simulink model "Tandem4Servers10000"  (R2023a)
settings: Solver=VariableStepAuto  StartTime=0.0  StopTime=100  RelTol=1e-3
undefined symbols (not defined in the file or in its folder): m, n
libraries: simulink x2
settings Model: PauseTimes=53  Creator=pratyaksh  LastModifiedBy=pratyaksh

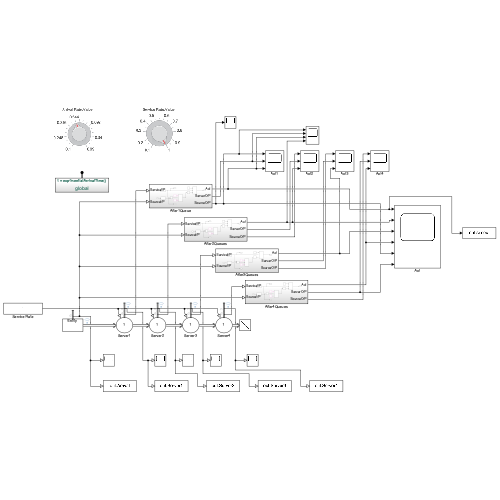
[thumbnail: Simulink's stored preview of the top-level diagram]
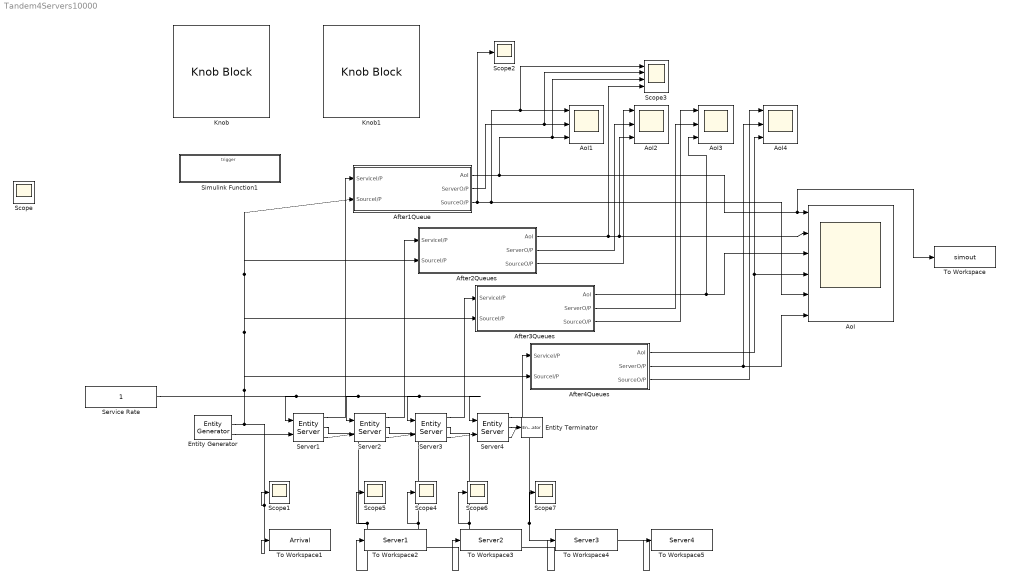
== system Tandem4Servers10000 ==
  After1Queue : Subsystem
  After2Queues : Subsystem
  After3Queues : Subsystem
  After4Queues : Subsystem
  AoI : Scope  NumInputPorts=6
  AoI{1..4} (4 alike) : Scope  NumInputPorts=3
  Entity Generator : EntityGenerator  OutputPortMessageModes=n,m  TimeSource=MATLAB action  Period=7  IntergenerationTimeAction=|  GenerateEntityAtSimulationStart=off  AttributeInitialValue=0  NumberEntitiesDeparted=on  EntityType=Structured  EntityTypeName=Entity
      | T = exponentialArrivalTime;   % fixed intergeneration time
      | N = 10000;   % number of entities generated
      | persistent nr;
      | if isempty(nr)
      |   nr = 1;
      | end
      | 
      | if nr <= N
      |   dt = T;
      | else
      |   dt = inf;
      | end
      | nr = nr + 1;
      settings: OutputPortMap=o0,o3
  Entity Terminator : EntityTerminator  InputPortMessageModes=m
  Knob : KnobBlock  ScaleMin=0.10000000000000001  ScaleMax=0.99
  Knob1 : KnobBlock  ScaleMin=0.10000000000000001  ScaleMax=1
  Scope{,1..2,4..7} (7 alike) : Scope
  Scope3 : Scope  NumInputPorts=4
  Server1 : EntityServer  InputPortMessageModes=n,m  OutputPortMessageModes=n,n,m  Capacity=1  ServiceTimeSource=Signal port  ServiceTimeAction=|  NumberEntitiesDeparted=on  NumberEntitiesInBlock=on
      | persistent rngInit;
      | if isempty(rngInit)
      |     seed = 12345;
      |     rng(seed);
      |     rngInit = true;
      | end
      | 
      | % Pattern: Exponential distribution
      | mu = 1;
      | dt = -mu * log(1 - rand());
      settings: InputPortMap=u0,u2  OutputPortMap=o0,o1,o9
  Server2 : EntityServer  InputPortMessageModes=n,m  OutputPortMessageModes=n,n,m  Capacity=1  ServiceTimeSource=Signal port  ServiceTimeAction=|  NumberEntitiesDeparted=on  NumberEntitiesInBlock=on
      | persistent rngInit;
      | if isempty(rngInit)
      |     seed = 12345;
      |     rng(seed);
      |     rngInit = true;
      | end
      | 
      | % Pattern: Exponential distribution
      | mu = 1;
      | dt = -mu * log(1 - rand());
      settings: InputPortMap=u0,u2  OutputPortMap=o0,o1,o9
  Server3 : EntityServer  InputPortMessageModes=n,m  OutputPortMessageModes=n,n,m  Capacity=1  ServiceTimeSource=Signal port  ServiceTimeAction=|  NumberEntitiesDeparted=on  NumberEntitiesInBlock=on
      | persistent rngInit;
      | if isempty(rngInit)
      |     seed = 12345;
      |     rng(seed);
      |     rngInit = true;
      | end
      | 
      | % Pattern: Exponential distribution
      | mu = 1;
      | dt = -mu * log(1 - rand());
      settings: InputPortMap=u0,u2  OutputPortMap=o0,o1,o9
  Server4 : EntityServer  InputPortMessageModes=n,m  OutputPortMessageModes=n,n,m  Capacity=1  ServiceTimeSource=Signal port  ServiceTimeAction=|  NumberEntitiesDeparted=on  NumberEntitiesInBlock=on
      | persistent rngInit;
      | if isempty(rngInit)
      |     seed = 12345;
      |     rng(seed);
      |     rngInit = true;
      | end
      | 
      | % Pattern: Exponential distribution
      | mu = 1;
      | dt = -mu * log(1 - rand());
      settings: InputPortMap=u0,u2  OutputPortMap=o0,o1,o9
  Service Rate : Constant  SampleTime=-1
  Simulink Function1 : Subsystem  TreatAsAtomicUnit=on
  To Workspace : ToWorkspace  VariableName=simout  SampleTime=-1
      settings: MaxDataPoints=2  Save2DSignal=2-D array (concatenate along first dimension)
  To Workspace1 : ToWorkspace  VariableName=Arrival  SaveFormat=Timeseries  SampleTime=-1
  To Workspace2 : ToWorkspace  VariableName=Server1  SaveFormat=Timeseries  SampleTime=-1
      settings: Save2DSignal=2-D array (concatenate along first dimension)
  To Workspace3 : ToWorkspace  VariableName=Server2  SaveFormat=Timeseries  SampleTime=-1
      settings: Save2DSignal=2-D array (concatenate along first dimension)
  To Workspace4 : ToWorkspace  VariableName=Server3  SaveFormat=Timeseries  SampleTime=-1
      settings: Save2DSignal=2-D array (concatenate along first dimension)
  To Workspace5 : ToWorkspace  VariableName=Server4  SaveFormat=Timeseries  SampleTime=-1
      settings: Save2DSignal=2-D array (concatenate along first dimension)
  wires:
  Service Rate/1 -> Server1/1, Server2/1, Server3/1, Server4/1
  Entity Generator/2 -> Server1/2
  Server3/3 -> Server4/2
  Server4/3 -> Entity Terminator/1
  Server1/3 -> Server2/2
  Server2/3 -> Server3/2
  Entity Generator/1 -> After4Queues/2(SourceI/P), After2Queues/2(SourceI/P), After1Queue/2(SourceI/P), After3Queues/2(SourceI/P), To Workspace1/1, Scope1/1
  Server4/1 -> After4Queues/1(ServiceI/P)
  Server3/1 -> After3Queues/1(ServiceI/P)
  Server2/1 -> After2Queues/1(ServiceI/P)
  Server1/1 -> After1Queue/1(ServiceI/P)
  After2Queues/1(AoI) -> Scope3/4, AoI/2, AoI2/3
  After3Queues/1(AoI) -> AoI/3, AoI3/3
  After4Queues/1(AoI) -> AoI4/3, AoI/4
  After1Queue/3(SourceO/P) -> Scope2/1, Scope3/1, AoI1/1, AoI/5
  After4Queues/2(ServerO/P) -> AoI/6, AoI4/2
  After1Queue/2(ServerO/P) -> Scope3/2, AoI1/2
  After2Queues/3(SourceO/P) -> AoI2/1
  After2Queues/2(ServerO/P) -> AoI2/2
  After3Queues/3(SourceO/P) -> AoI3/1
  After3Queues/2(ServerO/P) -> AoI3/2
  After4Queues/3(SourceO/P) -> AoI4/1
  After1Queue/1(AoI) -> Scope3/3, AoI1/3, To Workspace/1, AoI/1
  Server2/2 -> To Workspace3/1, Scope4/1
  Server3/2 -> To Workspace4/1, Scope6/1
  Server4/2 -> To Workspace5/1, Scope7/1
  Server1/2 -> To Workspace2/1, Scope5/1

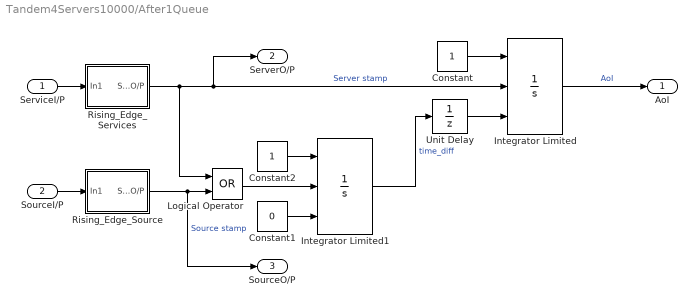
== system Tandem4Servers10000/After1Queue ==
  ServiceI/P : Inport
  SourceI/P : Inport  Port=2
  Constant : Constant
  Constant1 : Constant  Value=0
  Constant2 : Constant
  Integrator Limited : Integrator  ExternalReset=rising  InitialConditionSource=external  LimitOutput=on  UpperSaturationLimit=1000  LowerSaturationLimit=0
  Integrator Limited1 : Integrator  ExternalReset=rising  InitialConditionSource=external  LimitOutput=on  UpperSaturationLimit=1000  LowerSaturationLimit=0
  Logical Operator : Logic  Operator=OR  AllPortsSameDT=off  OutDataTypeStr=boolean
  Rising_Edge_Services : Subsystem
  Rising_Edge_Source : Subsystem
  Unit Delay : UnitDelay  SampleTime=-1  HasFrameUpgradeWarning=on
  AoI : Outport
  ServerO/P : Outport  Port=2
  SourceO/P : Outport  Port=3
  wires:
  Unit Delay/1 -> Integrator Limited/3
  Logical Operator/1 -> Integrator Limited1/2
  Rising_Edge_Source/1(SourceO/P) -> SourceO/P/1, Logical Operator/2  "Source stamp"
  Integrator Limited1/1 -> Unit Delay/1  "time_diff"
  Constant1/1 -> Integrator Limited1/3
  Rising_Edge_Services/1(ServerO/P) -> ServerO/P/1, Integrator Limited/2, Logical Operator/1  "Server stamp"
  Constant2/1 -> Integrator Limited1/1
  SourceI/P/1 -> Rising_Edge_Source/1(In1)
  ServiceI/P/1 -> Rising_Edge_Services/1(In1)
  Constant/1 -> Integrator Limited/1
  Integrator Limited/1 -> AoI/1  "AoI"

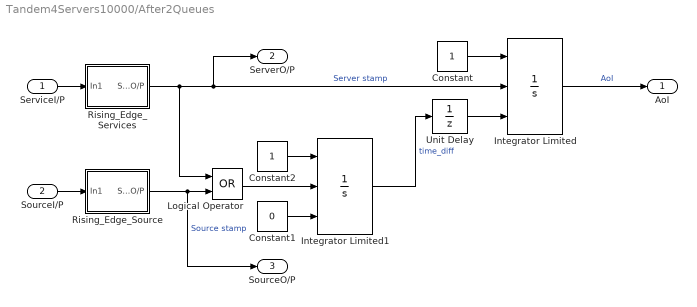
== system Tandem4Servers10000/After2Queues ==
  ServiceI/P : Inport
  SourceI/P : Inport  Port=2
  Constant : Constant
  Constant1 : Constant  Value=0
  Constant2 : Constant
  Integrator Limited : Integrator  ExternalReset=rising  InitialConditionSource=external  LimitOutput=on  UpperSaturationLimit=1000  LowerSaturationLimit=0
  Integrator Limited1 : Integrator  ExternalReset=rising  InitialConditionSource=external  LimitOutput=on  UpperSaturationLimit=1000  LowerSaturationLimit=0
  Logical Operator : Logic  Operator=OR  AllPortsSameDT=off  OutDataTypeStr=boolean
  Rising_Edge_Services : Subsystem
  Rising_Edge_Source : Subsystem
  Unit Delay : UnitDelay  SampleTime=-1  HasFrameUpgradeWarning=on
  AoI : Outport
  ServerO/P : Outport  Port=2
  SourceO/P : Outport  Port=3
  wires:
  Unit Delay/1 -> Integrator Limited/3
  Logical Operator/1 -> Integrator Limited1/2
  Rising_Edge_Source/1(SourceO/P) -> SourceO/P/1, Logical Operator/2  "Source stamp"
  Integrator Limited1/1 -> Unit Delay/1  "time_diff"
  Constant1/1 -> Integrator Limited1/3
  Rising_Edge_Services/1(ServerO/P) -> ServerO/P/1, Integrator Limited/2, Logical Operator/1  "Server stamp"
  Constant2/1 -> Integrator Limited1/1
  SourceI/P/1 -> Rising_Edge_Source/1(In1)
  ServiceI/P/1 -> Rising_Edge_Services/1(In1)
  Constant/1 -> Integrator Limited/1
  Integrator Limited/1 -> AoI/1  "AoI"

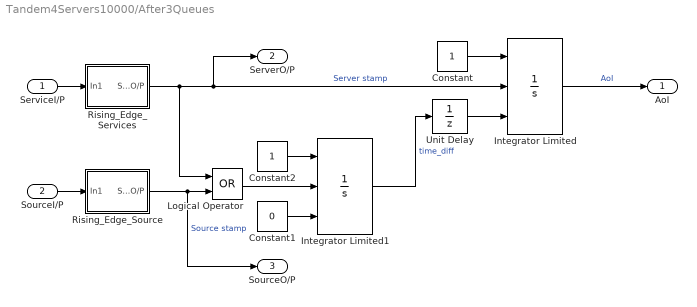
== system Tandem4Servers10000/After3Queues ==
  ServiceI/P : Inport
  SourceI/P : Inport  Port=2
  Constant : Constant
  Constant1 : Constant  Value=0
  Constant2 : Constant
  Integrator Limited : Integrator  ExternalReset=rising  InitialConditionSource=external  LimitOutput=on  UpperSaturationLimit=1000  LowerSaturationLimit=0
  Integrator Limited1 : Integrator  ExternalReset=rising  InitialConditionSource=external  LimitOutput=on  UpperSaturationLimit=1000  LowerSaturationLimit=0
  Logical Operator : Logic  Operator=OR  AllPortsSameDT=off  OutDataTypeStr=boolean
  Rising_Edge_Services : Subsystem
  Rising_Edge_Source : Subsystem
  Unit Delay : UnitDelay  SampleTime=-1  HasFrameUpgradeWarning=on
  AoI : Outport
  ServerO/P : Outport  Port=2
  SourceO/P : Outport  Port=3
  wires:
  Unit Delay/1 -> Integrator Limited/3
  Logical Operator/1 -> Integrator Limited1/2
  Rising_Edge_Source/1(SourceO/P) -> SourceO/P/1, Logical Operator/2  "Source stamp"
  Integrator Limited1/1 -> Unit Delay/1  "time_diff"
  Constant1/1 -> Integrator Limited1/3
  Rising_Edge_Services/1(ServerO/P) -> ServerO/P/1, Integrator Limited/2, Logical Operator/1  "Server stamp"
  Constant2/1 -> Integrator Limited1/1
  SourceI/P/1 -> Rising_Edge_Source/1(In1)
  ServiceI/P/1 -> Rising_Edge_Services/1(In1)
  Constant/1 -> Integrator Limited/1
  Integrator Limited/1 -> AoI/1  "AoI"

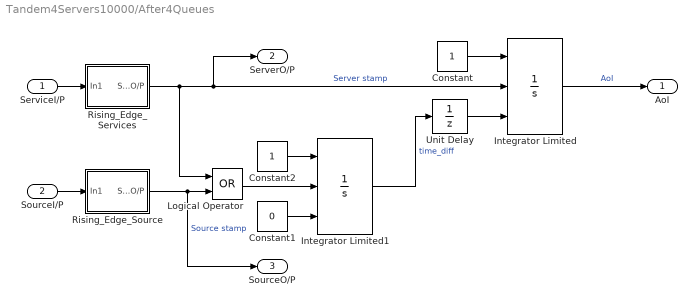
== system Tandem4Servers10000/After4Queues ==
  ServiceI/P : Inport
  SourceI/P : Inport  Port=2
  Constant : Constant
  Constant1 : Constant  Value=0
  Constant2 : Constant
  Integrator Limited : Integrator  ExternalReset=rising  InitialConditionSource=external  LimitOutput=on  UpperSaturationLimit=1000  LowerSaturationLimit=0
  Integrator Limited1 : Integrator  ExternalReset=rising  InitialConditionSource=external  LimitOutput=on  UpperSaturationLimit=1000  LowerSaturationLimit=0
  Logical Operator : Logic  Operator=OR  AllPortsSameDT=off  OutDataTypeStr=boolean
  Rising_Edge_Services : Subsystem
  Rising_Edge_Source : Subsystem
  Unit Delay : UnitDelay  SampleTime=-1  HasFrameUpgradeWarning=on
  AoI : Outport
  ServerO/P : Outport  Port=2
  SourceO/P : Outport  Port=3
  wires:
  Unit Delay/1 -> Integrator Limited/3
  Logical Operator/1 -> Integrator Limited1/2
  Rising_Edge_Source/1(SourceO/P) -> SourceO/P/1, Logical Operator/2  "Source stamp"
  Integrator Limited1/1 -> Unit Delay/1  "time_diff"
  Constant1/1 -> Integrator Limited1/3
  Rising_Edge_Services/1(ServerO/P) -> ServerO/P/1, Integrator Limited/2, Logical Operator/1  "Server stamp"
  Constant2/1 -> Integrator Limited1/1
  SourceI/P/1 -> Rising_Edge_Source/1(In1)
  ServiceI/P/1 -> Rising_Edge_Services/1(In1)
  Constant/1 -> Integrator Limited/1
  Integrator Limited/1 -> AoI/1  "AoI"

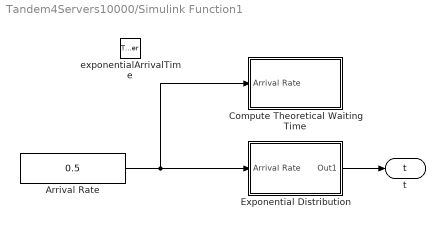
== system Tandem4Servers10000/Simulink Function1 ==
  exponentialArrivalTime : TriggerPort  TriggerType=function-call  IsSimulinkFunction=on  FunctionName=exponentialArrivalTime  VariantControl=Variant
  Arrival Rate : Constant  Value=0.5  SampleTime=-1
  Compute Theoretical Waiting Time : Subsystem
  Exponential Distribution : Subsystem
  t : ArgOut  DisableCoverage=on  ArgumentName=t
  wires:
  Exponential Distribution/1(Out1) -> t/1
  Arrival Rate/1 -> Exponential Distribution/1(Arrival Rate), Compute Theoretical Waiting Time/1(Arrival Rate)

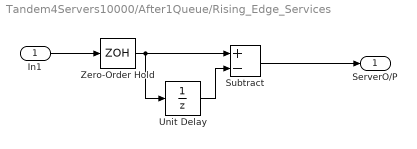
== system Tandem4Servers10000/After1Queue/Rising_Edge_Services ==
  In1 : Inport
  Subtract : Sum  Inputs=+-
  Unit Delay : UnitDelay  SampleTime=-1  HasFrameUpgradeWarning=on
  Zero-Order Hold : ZeroOrderHold  SampleTime=0.005
  ServerO/P : Outport  VectorParamsAs1DForOutWhenUnconnected=off
  wires:
  Zero-Order Hold/1 -> Unit Delay/1, Subtract/1
  Unit Delay/1 -> Subtract/2
  In1/1 -> Zero-Order Hold/1
  Subtract/1 -> ServerO/P/1

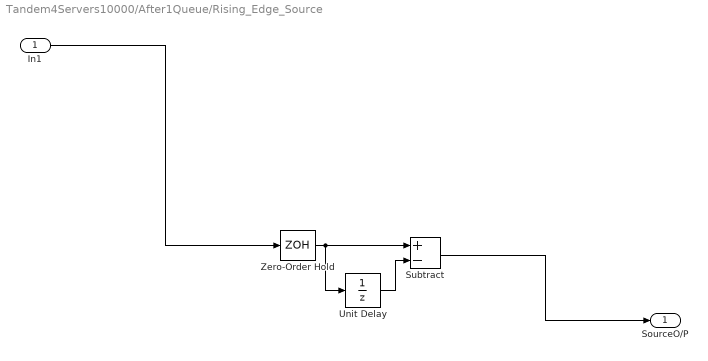
== system Tandem4Servers10000/After1Queue/Rising_Edge_Source ==
  In1 : Inport
  Subtract : Sum  Inputs=+-
  Unit Delay : UnitDelay  SampleTime=-1  HasFrameUpgradeWarning=on
  Zero-Order Hold : ZeroOrderHold  SampleTime=0.005
  SourceO/P : Outport  VectorParamsAs1DForOutWhenUnconnected=off
  wires:
  Zero-Order Hold/1 -> Unit Delay/1, Subtract/1
  Unit Delay/1 -> Subtract/2
  In1/1 -> Zero-Order Hold/1
  Subtract/1 -> SourceO/P/1

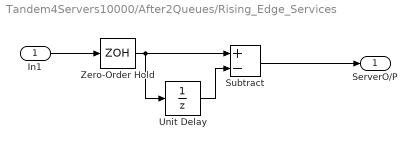
== system Tandem4Servers10000/After2Queues/Rising_Edge_Services ==
  In1 : Inport
  Subtract : Sum  Inputs=+-
  Unit Delay : UnitDelay  SampleTime=-1  HasFrameUpgradeWarning=on
  Zero-Order Hold : ZeroOrderHold  SampleTime=0.005
  ServerO/P : Outport  VectorParamsAs1DForOutWhenUnconnected=off
  wires:
  Zero-Order Hold/1 -> Unit Delay/1, Subtract/1
  Unit Delay/1 -> Subtract/2
  In1/1 -> Zero-Order Hold/1
  Subtract/1 -> ServerO/P/1

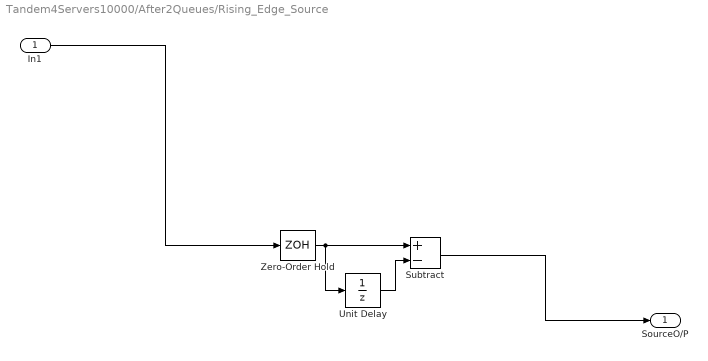
== system Tandem4Servers10000/After2Queues/Rising_Edge_Source ==
  In1 : Inport
  Subtract : Sum  Inputs=+-
  Unit Delay : UnitDelay  SampleTime=-1  HasFrameUpgradeWarning=on
  Zero-Order Hold : ZeroOrderHold  SampleTime=0.005
  SourceO/P : Outport  VectorParamsAs1DForOutWhenUnconnected=off
  wires:
  Zero-Order Hold/1 -> Unit Delay/1, Subtract/1
  Unit Delay/1 -> Subtract/2
  In1/1 -> Zero-Order Hold/1
  Subtract/1 -> SourceO/P/1

== system Tandem4Servers10000/After3Queues/Rising_Edge_Services ==
  In1 : Inport
  Subtract : Sum  Inputs=+-
  Unit Delay : UnitDelay  SampleTime=-1  HasFrameUpgradeWarning=on
  Zero-Order Hold : ZeroOrderHold  SampleTime=0.005
  ServerO/P : Outport  VectorParamsAs1DForOutWhenUnconnected=off
  wires:
  Zero-Order Hold/1 -> Unit Delay/1, Subtract/1
  Unit Delay/1 -> Subtract/2
  In1/1 -> Zero-Order Hold/1
  Subtract/1 -> ServerO/P/1

== system Tandem4Servers10000/After3Queues/Rising_Edge_Source ==
  In1 : Inport
  Subtract : Sum  Inputs=+-
  Unit Delay : UnitDelay  SampleTime=-1  HasFrameUpgradeWarning=on
  Zero-Order Hold : ZeroOrderHold  SampleTime=0.005
  SourceO/P : Outport  VectorParamsAs1DForOutWhenUnconnected=off
  wires:
  Zero-Order Hold/1 -> Unit Delay/1, Subtract/1
  Unit Delay/1 -> Subtract/2
  In1/1 -> Zero-Order Hold/1
  Subtract/1 -> SourceO/P/1

== system Tandem4Servers10000/After4Queues/Rising_Edge_Services ==
  In1 : Inport
  Subtract : Sum  Inputs=+-
  Unit Delay : UnitDelay  SampleTime=-1  HasFrameUpgradeWarning=on
  Zero-Order Hold : ZeroOrderHold  SampleTime=0.005
  ServerO/P : Outport  VectorParamsAs1DForOutWhenUnconnected=off
  wires:
  Zero-Order Hold/1 -> Unit Delay/1, Subtract/1
  Unit Delay/1 -> Subtract/2
  In1/1 -> Zero-Order Hold/1
  Subtract/1 -> ServerO/P/1

== system Tandem4Servers10000/After4Queues/Rising_Edge_Source ==
  In1 : Inport
  Subtract : Sum  Inputs=+-
  Unit Delay : UnitDelay  SampleTime=-1  HasFrameUpgradeWarning=on
  Zero-Order Hold : ZeroOrderHold  SampleTime=0.005
  SourceO/P : Outport  VectorParamsAs1DForOutWhenUnconnected=off
  wires:
  Zero-Order Hold/1 -> Unit Delay/1, Subtract/1
  Unit Delay/1 -> Subtract/2
  In1/1 -> Zero-Order Hold/1
  Subtract/1 -> SourceO/P/1

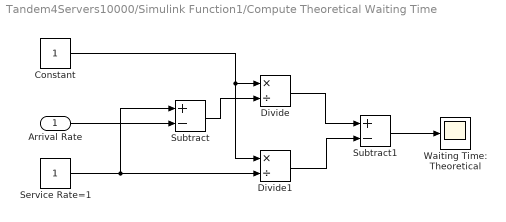
== system Tandem4Servers10000/Simulink Function1/Compute Theoretical Waiting Time ==
  Arrival Rate : Inport
  Constant : Constant
  Divide : Product  Inputs=*/
  Divide1 : Product  Inputs=*/
  Service Rate=1 : Constant
  Subtract : Sum  Inputs=+-
  Subtract1 : Sum  Inputs=+-
  Waiting Time: Theoretical : Scope
  wires:
  Service Rate=1/1 -> Divide1/2, Subtract/1
  Constant/1 -> Divide/1, Divide1/1
  Subtract/1 -> Divide/2
  Divide/1 -> Subtract1/1
  Divide1/1 -> Subtract1/2
  Subtract1/1 -> Waiting Time: Theoretical/1
  Arrival Rate/1 -> Subtract/2

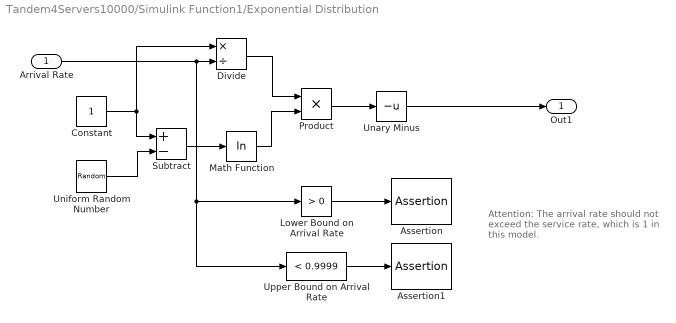
== system Tandem4Servers10000/Simulink Function1/Exponential Distribution ==
  note: Attention: The arrival rate
      | should not exceed the service
      | rate, which is 1 in this model.
  Arrival Rate : Inport
  Assertion : Assertion
  Assertion1 : Assertion
  Constant : Constant
  Divide : Product  Inputs=*/
  Lower Bound on Arrival Rate : simulink/Logic and Bit Operations/Compare To Constant  relop=>  const=0  OutDataTypeStr=uint8  ZeroCross=off
  Math Function : Math  Operator=log  SignedPower=on
  Product : Product  RndMeth=Zero
  Subtract : Sum  Inputs=+-
  Unary Minus : UnaryMinus
  Uniform Random Number : UniformRandomNumber  Minimum=0  Seed=12345
  "Upper Bound on Arrival Rate " : simulink/Logic and Bit Operations/Compare To Constant  relop=<  const=0.9999  OutDataTypeStr=uint8  ZeroCross=off
  Out1 : Outport  VectorParamsAs1DForOutWhenUnconnected=off
  wires:
  Subtract/1 -> Math Function/1
  "Upper Bound on Arrival Rate "/1 -> Assertion1/1
  Lower Bound on Arrival Rate/1 -> Assertion/1
  Uniform Random Number/1 -> Subtract/2
  Constant/1 -> Subtract/1, Divide/1
  Divide/1 -> Product/1
  Math Function/1 -> Product/2
  Product/1 -> Unary Minus/1
  Unary Minus/1 -> Out1/1
  Arrival Rate/1 -> "Upper Bound on Arrival Rate "/1, Lower Bound on Arrival Rate/1, Divide/2
